simulink model "land_detector"  (R2021a)
settings: Solver=FixedStepAuto  StartTime=0.0  StopTime=10.0  FixedStep=0.04  RelTol=1e-3
undefined symbols (not defined in the file): LNDFW_AIRSPD_MAX, LNDFW_VEL_XY_MAX, LNDFW_VEL_Z_MAX, LNDFW_XYACC_MAX, LNDMC_ALT_GND, LNDMC_ROT_MAX, LNDMC_XY_VEL_MAX, LNDMC_Z_VEL_MAX, MPC_LAND_SPEED, MPC_MANTHR_MIN, MPC_THR_HOVER, MPC_THR_MIN
settings Model: DataDictionary=px4_dict.sldd  Creator=DELL  LastModifiedBy=DELL
settings OptimizationCC: DefaultUnderspecifiedDataType=single

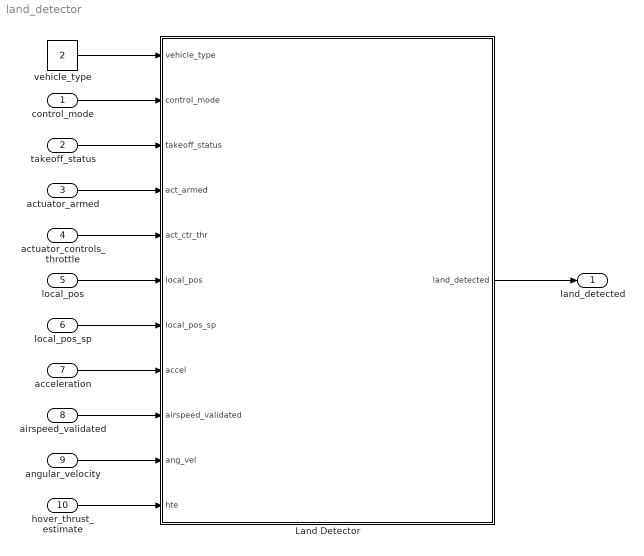
== system land_detector ==
  control_mode : Inport  OutDataTypeStr=Bus: px4_vehicle_control_mode
  takeoff_status : Inport  Port=2  OutDataTypeStr=Bus: px4_takeoff_status
  actuator_armed : Inport  Port=3  OutDataTypeStr=Bus: px4_actuator_armed
  actuator_controls_throttle : Inport  Port=4  OutDataTypeStr=Bus: px4_actuator_controls
  local_pos : Inport  Port=5  OutDataTypeStr=Bus: px4_vehicle_local_position
  local_pos_sp : Inport  Port=6  OutDataTypeStr=Bus: px4_vehicle_local_position_setpoint
  acceleration : Inport  Port=7  OutDataTypeStr=Bus: px4_vehicle_acceleration
  airspeed_validated : Inport  Port=8  OutDataTypeStr=Bus: px4_airspeed_validated
  angular_velocity : Inport  Port=9  OutDataTypeStr=Bus: px4_vehicle_angular_velocity
  hover_thrust_estimate : Inport  Port=10  OutDataTypeStr=Bus: px4_hover_thrust_estimate
  Land Detector : Stateflow chart  TreatAsAtomicUnit=on
  vehicle_type : Constant  Value=2  OutDataTypeStr=uint8
  land_detected : Outport
  wires:
  hover_thrust_estimate/1 -> Land Detector/11(hte)
  takeoff_status/1 -> Land Detector/3(takeoff_status)
  local_pos/1 -> Land Detector/6(local_pos)
  acceleration/1 -> Land Detector/8(accel)
  Land Detector/1(land_detected) -> land_detected/1
  control_mode/1 -> Land Detector/2(control_mode)
  local_pos_sp/1 -> Land Detector/7(local_pos_sp)
  vehicle_type/1 -> Land Detector/1(vehicle_type)
  airspeed_validated/1 -> Land Detector/9(airspeed_validated)
  actuator_armed/1 -> Land Detector/4(act_armed)
  actuator_controls_throttle/1 -> Land Detector/5(act_ctr_thr)
  angular_velocity/1 -> Land Detector/10(ang_vel)

== stateflow chart land_detector/Land Detector ==
  state Land_Logical [parallel]
    settings: executionOrder=1
    state mc
      state freefall [parallel]
        settings: executionOrder=1
        state freefall_true
          en,du:
          freefall_state_ = true;
        state freefall_false
          en,du:
          freefall_state_ = false;
        (default) -> Land_Logical.mc.freefall.freefall_true
        Land_Logical.mc.freefall.freefall_true -> Land_Logical.mc.freefall.freefall_false : [duration(get_freefall_state(accel.xyz)) > 0.03]
        Land_Logical.mc.freefall.freefall_false -> Land_Logical.mc.freefall.freefall_true : [duration(~get_freefall_state(accel.xyz)) > 0.03]
      state ground_contact [parallel]
        en,du:
        [vertical_movement_state_, ...
        horizontal_movement_state_, ...
        ground_contact_state_, ...
        in_descend_state_, ...
        close_to_ground_or_skipped_check_state_, ...
        alt_max_] = ...
        get_ground_contact_state;
        settings: executionOrder=2
      state maybe_land [parallel]
        en,du:
        low_throttle_state_ = is_low_throttle(maybe_landed_state_);
        settings: executionOrder=3
        state maybe_land_true
          en,du:
          maybe_landed_state_ = true;
        state maybe_land_false
          en,du:
          maybe_landed_state_ = false;
        (default) -> Land_Logical.mc.maybe_land.maybe_land_true
        Land_Logical.mc.maybe_land.maybe_land_true -> Land_Logical.mc.maybe_land.maybe_land_false : [act_armed.armed || ...
            | ~is_rotate]
        Land_Logical.mc.maybe_land.maybe_land_false -> Land_Logical.mc.maybe_land.maybe_land_true : [~act_armed.armed || ...
            | freefall_state_ || ...
            | (min_thrust_start > 0 && duration(low_throttle_state_)) > 8.0 || ...
            | freefall_state_ ||...
            | is_rotate]
      state landed [parallel]
        en,du:
        % reset the landed_time
        if (~maybe_landed_state_)
        landed_time_ = 0;
        elseif (landed_time_ == 0)
        landed_time_ = uint64(getSimulationTime);
        end
        % update in_ground_effect_state_
        in_ground_effect_state_ = (in_descend_state_ && horizontal_movement_state_) || ...
        (below_gnd_effect_hgt_state_ && takeoff_status.takeoff_state == uint8(PX4_TAKEOFF_STATUS.TAKEOFF_STATE_FLIGHT)) || ...
        takeoff_status.takeoff_state == uint8(PX4_TAKEOFF_STATUS.TAKEOFF_STATE_RAMPUP);
        settings: executionOrder=4
        state landed_true
          en,du:
          landed_state_ = true;
        state landed_false
          en,du:
          landed_state_ = false;
        (default) -> Land_Logical.mc.landed.landed_true
        Land_Logical.mc.landed.landed_true -> Land_Logical.mc.landed.landed_false : [act_armed.armed]
        Land_Logical.mc.landed.landed_false -> Land_Logical.mc.landed.landed_true : [~act_armed.armed]
    state vtol
      state freefall [parallel]
        settings: executionOrder=1
        state freefall_true
          en,du:
          freefall_state_ = true;
        state freefall_false
          en,du:
          freefall_state_ = false;
        (default) -> Land_Logical.vtol.freefall.freefall_true
        Land_Logical.vtol.freefall.freefall_true -> Land_Logical.vtol.freefall.freefall_false : [duration(get_freefall_state(accel.xyz)) > 0.03]
        Land_Logical.vtol.freefall.freefall_false -> Land_Logical.vtol.freefall.freefall_true : [duration(~get_freefall_state(accel.xyz)) > 0.03]
      state maybe_land [parallel]
        en,du:
        low_throttle_state_ = mc.maybe_land.is_low_throttle(maybe_landed_state_);
        maybe_landed_state_ = mc.maybe_land.is_rotate;
        settings: executionOrder=2
        state maybe_land_true
          en,du:
          maybe_landed_state_ = true;
        state maybe_land_false
          en,du:
          maybe_landed_state_ = false;
        (default) -> Land_Logical.vtol.maybe_land.maybe_land_true
        Land_Logical.vtol.maybe_land.maybe_land_true -> Land_Logical.vtol.maybe_land.maybe_land_false : [act_armed.armed]
        Land_Logical.vtol.maybe_land.maybe_land_false -> Land_Logical.vtol.maybe_land.maybe_land_true : [~act_armed.armed || ...
            | freefall_state_ || ...
            | (min_thrust_start > 0 && duration(low_throttle_state_)) > 8.0 || ...
            | freefall_state_]
      state landed [parallel]
        en,du:
        % reset the landed_time
        if (~maybe_landed_state_)
        landed_time_ = 0;
        elseif (landed_time_ == 0)
        landed_time_ = uint64(getSimulationTime);
        end
        % update in_ground_effect_state_
        in_ground_effect_state_ = (in_descend_state_ && horizontal_movement_state_) || ...
        (below_gnd_effect_hgt_state_ && takeoff_status.takeoff_state == uint8(PX4_TAKEOFF_STATUS.TAKEOFF_STATE_FLIGHT)) || ...
        takeoff_status.takeoff_state == uint8(PX4_TAKEOFF_STATUS.TAKEOFF_STATE_RAMPUP);
        % airspeed filtered
        if ((uint64(getSimulationTime) * 1000 - airspeed_validated.timestamp < 1000) && isfinite(airspeed_validated.true_airspeed_m_s))
        airspeed_filtered = single(0.95 * airspeed_filtered + 0.05 * airspeed_validated.true_airspeed_m_s);
        else
        % if airspeed does not update, set it to zero and rely on multicopter land detector
        airspeed_filtered = single(0.0);
        end
        settings: executionOrder=3
        state landed_true
          en,du:
          landed_state_ = true;
        state landed_false
          en,du:
          landed_state_ = false;
        (default) -> Land_Logical.vtol.landed.landed_true
        Land_Logical.vtol.landed.landed_true -> Land_Logical.vtol.landed.landed_false : [act_armed.armed || ...
            | (airspeed_filtered  > LNDFW_AIRSPD_MAX)]
        Land_Logical.vtol.landed.landed_false -> Land_Logical.vtol.landed.landed_true : [~act_armed.armed]
    state fw
      state landed_true
        en,du:
        landed_state_ = true;
      state landed_false
        en,du:
        landed_state_ = fw_land_detected;
      (default) -> Land_Logical.fw.landed_true
      Land_Logical.fw.landed_true -> Land_Logical.fw.landed_false : [uint64(getSimulationTime) * 1000 - local_pos.timestamp < 1000]
      Land_Logical.fw.landed_false -> Land_Logical.fw.landed_true : [~act_armed.armed || ...
          | uint64(getSimulationTime) * 1000 - local_pos.timestamp > 1000]
    (default) -> (junction 23)
    (junction 23) -> mc [order 1] : [vehicle_type == 1]
    (junction 23) -> (junction 25) [order 2]
    (junction 25) -> vtol [order 1] : [vehicle_type == 2]
    (junction 25) -> (junction 28) [order 2]
    (junction 28) -> fw
  state Publish_Data [parallel]
    en,du:
    land_detected.timestamp = uint64(getSimulationTime);
    land_detected.freefall = freefall_state_;
    land_detected.ground_contact = ground_contact_state_;
    land_detected.maybe_landed = maybe_landed_state_;
    land_detected.landed = landed_state_;
    land_detected.alt_max = alt_max_;
    land_detected.in_ground_effect = in_ground_effect_state_;
    land_detected.in_descend = in_descend_state_;
    land_detected.has_low_throttle = low_throttle_state_;
    land_detected.horizontal_movement = horizontal_movement_state_;
    land_detected.vertical_movement = vertical_movement_state_;
    land_detected.close_to_ground_or_skipped_check = close_to_ground_or_skipped_check_state_;
    settings: executionOrder=2
  data: state function_output size=1; accel_xyz function_input; ver_move function_output; horiz_move function_output; gnd_contact function_output; in_descend function_output; close_to_ground_or_skipped_check function_output; gnd_effect_altitude function_output; state function_output; last_state function_input; state function_output; min_thrust_start local uint64 size=1 =uint64(0); min_thrust_start local uint64 size=1 =uint64(0); airspeed_filtered local single size=1 =single(0.0); land_state function_output; velocity_xy_filtered local single size=1 =single(0.0); velocity_z_filtered local single size=1 =single(0.0); airspeed_filtered local single size=1 =single(0.0); xy_accel_filtered local single size=1 =single(0.0); LNDFW_VEL_XY_MAX parameter; LNDFW_VEL_Z_MAX parameter; LNDFW_XYACC_MAX parameter; MPC_MANTHR_MIN parameter; MPC_THR_HOVER parameter; MPC_LAND_SPEED parameter; LNDMC_Z_VEL_MAX parameter; LNDMC_XY_VEL_MAX parameter; LNDMC_ALT_GND parameter; MPC_THR_MIN parameter; LNDMC_ROT_MAX parameter; LNDFW_AIRSPD_MAX parameter; vehicle_type input uint8 size=1; control_mode input Bus: px4_vehicle_control_mode size=1; takeoff_status input Bus: px4_takeoff_status size=1; act_armed input Bus: px4_actuator_armed size=1; act_ctr_thr input Bus: px4_actuator_controls size=1; land_detected output Bus: px4_vehicle_land_detected size=1; local_pos input Bus: px4_vehicle_local_position size=1; local_pos_sp input Bus: px4_vehicle_local_position_setpoint size=1; accel input Bus: px4_vehicle_acceleration size=1; landed_time_ local uint64 size=1 =uint64(0); vertical_movement_state_ local boolean size=1 =false; horizontal_movement_state_ local boolean size=1 =false; ground_contact_state_ local boolean size=1 =false; freefall_state_ local boolean size=1 =false; in_descend_state_ local boolean size=1 =false; maybe_landed_state_ local boolean size=1 =true; landed_state_ local boolean size=1 =true; close_to_ground_or_skipped_check_state_ local boolean size=1 =false; low_throttle_state_ local boolean size=1 =false; below_gnd_effect_hgt_state_ local boolean size=1 =false; in_ground_effect_state_ local boolean size=1 =false; alt_max_ local single size=1 =single(inf); airspeed_validated input Bus: px4_airspeed_validated size=1; ang_vel input Bus: px4_vehicle_angular_velocity size=1; hte input Bus: px4_hover_thrust_estimate size=1
  function state = get_freefall_state(accel_xyz):
    | function state = get_freefall_state(accel_xyz)
    | 
    | if(norm(accel_xyz) < 2.0)
    |     state = true;
    | else
    |     state = false;
    | end
    | 
    | end
  function [ver_move, horiz_move, ...:
    | function [ver_move, horiz_move, ...
    |     gnd_contact, in_descend, ...
    |     close_to_ground_or_skipped_check, ...
    |     gnd_effect_altitude] = get_ground_contact_state
    | 
    | time_now_us = uint64(getSimulationTime);
    | 
    | % 默认保持上一拍值
    | ground_contact = ground_contact_state_;
    | close_to_ground_or_skipped_check = close_to_ground_or_skipped_check_state_;
    | 
    | % 判断local_pos数据与当前时间间隔是否大于1s，如果大于1s，那么local_pos数据不可用
    | if ((time_now_us * 1000 - local_pos.timestamp) < 1000)
    |     lpos_available = true;
    | else
    |     lpos_available = false;
    | end
    | 
    | % land speed threshold, 90% of MPC_LAND_SPEED
    | % MPC_LAND_SPEED 多旋翼默认下降速度 0.7m/s
    | land_speed_threshold = 0.9 * max(MPC_LAND_SPEED, 0.1);
    | 
    | %% 垂直方向的运动检测
    | ver_move = false;
    | if (lpos_available && local_pos.v_z_valid)
    |     % Check if we are moving vertically - this might see a spike after arming due to
    |     % throttle-up vibration. If accelerating fast the throttle thresholds will still give
    |     % an accurate in-air indication.
    |     max_climb_rate = min(land_speed_threshold * 0.5, MPC_LAND_SPEED);
    |     % 在下降落地的2s内，将检测的阈值放大2.5倍
    |     if ((time_now_us - landed_time_) < 2)
    |         % Widen acceptance thresholds for landed state right after arming
    |         % so that motor spool-up and other effects do not trigger false negatives.
    |         % LNDMC_Z_VEL_MAX 多旋翼在下降过程中，在垂直方向上允许的最大速度，默认0.5m/s
    |         max_climb_rate = LNDMC_Z_VEL_MAX * 2.5;
    |         ver_move = abs(local_pos.vz) > max_climb_rate;
    |     else
    |         ver_move = false;
    |     end
    | end
    | 
    | %% 水平方向的运动检测
    | % 在下降过程中，水平方向的速度阈值为LNDMC_XY_VEL_MAX，1.5m/s
    | if (lpos_available && local_pos.v_xy_valid)
    |     v_xy = [local_pos.vx, local_pos.vy];
    |     horiz_move = norm(v_xy) > LNDMC_XY_VEL_MAX;
    | else
    |     horiz_move = false; % 由于local_pos数据无效，暂时还不确定水平方向有没有运动
    | end
    | 
    | %% 飞机是否在产生地效的高度以下
    | % LNDMC_ALT_GND默认为-1，无地效高度使用
    | if(LNDMC_ALT_GND < 0.0)
    |     gnd_effect_altitude = single(inf);
    | else
    |     gnd_effect_altitude = single(LNDMC_ALT_GND);
    | end
    | 
    | if (lpos_available && local_pos.dist_bottom_valid)
    |     below_gnd_effect_hgt_state_ = local_pos.dist_bottom < gnd_effect_altitude;
    | else
    |     below_gnd_effect_hgt_state_ = false;
    | end
    | 
    | %% 判断盘旋推力的有效性
    | hover_thrust_estimate_valid = (time_now_us - hte.timestamp) < 1;
    | 
    | % low thrust: 30% of throttle range between min and hover, relaxed to 60% if hover thrust estimate available
    | % 最小和悬停之间30%的油门范围属于低推力的范围，如果悬停推力估计可用，放宽到60%
    | if (hover_thrust_estimate_valid)
    |     thr_pct_hover = 0.6;
    | else
    |     thr_pct_hover = 0.3;
    | end
    | 
    | % MPC_THR_MIN 多旋翼下降过程中的最小油门，默认0.12
    | % MPC_THR_HOVER 多旋翼盘旋的油门，默认.05
    | sys_low_throttle = MPC_THR_MIN + (MPC_THR_HOVER - MPC_THR_MIN) * thr_pct_hover;
    | gnd_contact = act_ctr_thr.control(3) <= sys_low_throttle;
    | 
    | %% 判断飞机是不是在下降
    | % if we have a valid velocity setpoint and the vehicle is demanded to go down but no vertical movement present,
    | % we then can assume that the vehicle hit ground
    | 
    | % 默认保持上一拍的状态
    | in_descend = in_descend_state_;
    | 
    | if (control_mode.flag_control_climb_rate_enabled)
    |     
    |     % Setpoints can be nan
    |     in_descend = isfinite(local_pos_sp.vz) &&  (local_pos_sp.vz >= land_speed_threshold);
    |     
    |     % ground contact requires commanded descent until landed
    |     % 地面接触要求降落,直到着陆
    |     % 确定在着陆状态下才判断ground_contact
    |     if (~maybe_landed_state_ && ~landed_state_)
    |         ground_contact = ground_contact_state_ & in_descend_state_;
    |     else
    |         in_descend = false; 
    |     end
    |     
    |     %% 对地检测
    |     % if there is no distance to ground estimate available then don't enforce using it.
    | 	% if a distance to the ground estimate is generally available (_dist_bottom_is_observable=true), then
    | 	% we already increased the hysteresis for the land detection states in order to reduce the chance of false positives.
    |     
    |     % 判断飞机是不是接近地面在1m以内，需要down的数据有效
    |     if (local_pos.dist_bottom_valid)
    | 		is_close_to_ground = local_pos.dist_bottom < 1;
    | 	else
    | 		is_close_to_ground = false;
    |     end
    | 	
    |     % 无下视数据或者数据无效，跳过检测
    |     dist_bottom_is_observable = uint8(local_pos.dist_bottom_sensor_bitfield);
    |     dist_bottom_is_observable = bitand(dist_bottom_is_observable,0b0010);
    | 	skip_close_to_ground_check = ~dist_bottom_is_observable || ~local_pos.dist_bottom_valid;
    | 	close_to_ground_or_skipped_check = is_close_to_ground || skip_close_to_ground_check;
    | 
    | 	% When not armed, consider to have ground-contact
    |     % 如果没有解锁，那就与地面有接触
    | 	if (~act_armed.armed) 
    | 		gnd_contact = true;
    |     end
    |     
    |    % TODO: we need an accelerometer based check for vertical movement for flying without GPS
    |    % 如果没有gps, 需要使用加计来确定是否在垂直有运动
    | 	ground_contact = close_to_ground_or_skipped_check && ground_contact && ~horiz_move && ~ver_move;
    |     
    | end
  function state = is_low_throttle(last_state):
    | function state = is_low_throttle(last_state)
    | 
    | % 先保持上一拍的值
    | state = last_state;
    | 
    | % minimal throttle: initially 10% of throttle range between min and hover
    | % MPC_THR_MIN 多旋翼自动模式下得最小油门，默认0.12
    | % MPC_THR_HOVER 多旋翼悬停油门，默认0.5
    | sys_min_throttle = MPC_THR_MIN + (MPC_THR_HOVER - MPC_THR_MIN) * 0.1;
    | 
    | % Determine the system min throttle based on flight mode
    | % MPC_MANTHR_MIN 多旋翼垂直方向最小油门，默认0.01
    | if (~control_mode.flag_control_climb_rate_enabled)
    |     sys_min_throttle = (MPC_MANTHR_MIN + 0.01);
    | end
    | 
    | % Check if thrust output is less than the minimum throttle
    | if (act_ctr_thr.control(3) < sys_min_throttle)
    |     
    |     if (min_thrust_start == uint64(0))
    |         min_thrust_start = uint64(getSimulationTime);
    |         state = true;
    |     else
    |         min_thrust_start = uint64(0);
    |         state = false;
    |     end
    |     
    | end
    | 
    | end
  function state = is_rotate:
    | function state = is_rotate
    | 
    | state = maybe_landed_state_;
    | time_now_us = uint64(getSimulationTime);
    | landThresholdFactor = 1.0;
    | 
    | % Widen acceptance thresholds for landed state right after landed
    | if ((time_now_us - landed_time_) < 2)
    |     landThresholdFactor = 2.5;
    | end
    | 
    | % Next look if all rotation angles are not moving.
    | angular_velocity = [ang_vel.xyz(1), ang_vel.xyz(2)];
    | max_rotation_scaled = deg2rad(LNDMC_ROT_MAX) * landThresholdFactor;
    | 
    | if (norm(angular_velocity) > max_rotation_scaled)
    |     state = false;
    | end
    | 
    | % If vertical velocity is available: ground contact, no thrust, no movement -> landed
    | if (((time_now_us - local_pos.timestamp) < 1000) && local_pos.v_z_valid)
    |     [vertical_movement_state_, ...
    |         horizontal_movement_state_, ...
    |         ground_contact_state_, ...
    |         in_descend_state_, ...
    |         close_to_ground_or_skipped_check_state_] = ground_contact.get_ground_contact_state;
    | end
    | 
    | end
  function land_state = fw_land_detected:
    | function land_state = fw_land_detected
    | 
    | land_state = landed_state_;
    | 
    | % Horizontal velocity complimentary filter.
    | val = single(0.97 * velocity_xy_filtered + 0.03 * sqrt(local_pos.vx * local_pos.vx + local_pos.vy * local_pos.vy));
    | 
    | if (isfinite(val))
    |     velocity_xy_filtered = val;
    | end
    | 
    | % Vertical velocity complimentary filter.
    | val = single(0.99 * velocity_z_filtered + 0.01 * abs(local_pos.vz));
    | 
    | if (isfinite(val))
    |     velocity_z_filtered = val;
    | end
    | 
    | % set _airspeed_filtered to 0 if airspeed data is invalid
    | if (~isfinite(airspeed_validated.true_airspeed_m_s) || (uint64(getSimulationTime) * 1000 - airspeed_validated.timestamp) > 1000)
    |     airspeed_filtered = single(0.0);
    |     
    | else
    |     airspeed_filtered = single(0.95 * airspeed_filtered + 0.05 * airspeed_validated.true_airspeed_m_s);
    | end
    | 
    | % A leaking lowpass prevents biases from building up, but
    | % gives a mostly correct response for short impulses.
    | acc_hor = single(norm([accel.xyz(1), accel.xyz(2)])); % 水平加速度的模长
    | xy_accel_filtered = single(xy_accel_filtered * 0.8 + acc_hor * 0.18);
    | 
    | % Crude land detector for fixedwing.
    | land_state = ((airspeed_filtered < LNDFW_AIRSPD_MAX) && (velocity_xy_filtered < LNDFW_VEL_XY_MAX) && ...
    |     (velocity_z_filtered < LNDFW_VEL_Z_MAX) && (xy_accel_filtered < LNDFW_XYACC_MAX));
    | 
    | end
